simulink model "DSB_LC"  (R2024a)
settings: Solver=VariableStepAuto  StartTime=0.0  StopTime=10.0  RelTol=1e-3
libraries: dspfdesign x1
settings Model: Creator=mohamed
settings SolverCC: AlgebraicLoopSolver=TrustRegion
settings DebuggingCC: UnconnectedInputMsg=warning  UnconnectedOutputMsg=warning  UnconnectedLineMsg=warning
settings ModelReferenceCC: EnableRefExpFcnMdlSchedulingChecks=on
settings SFSimCC: CustomCodeUndefinedFunction=UseInterfaceOnly
settings RTWCC: GPUComputeCapability=3.5  DLArmComputeVersion=19.05

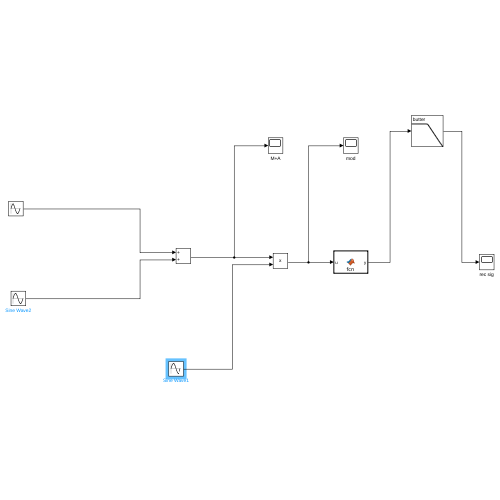
[thumbnail: Simulink's stored preview of the top-level diagram]
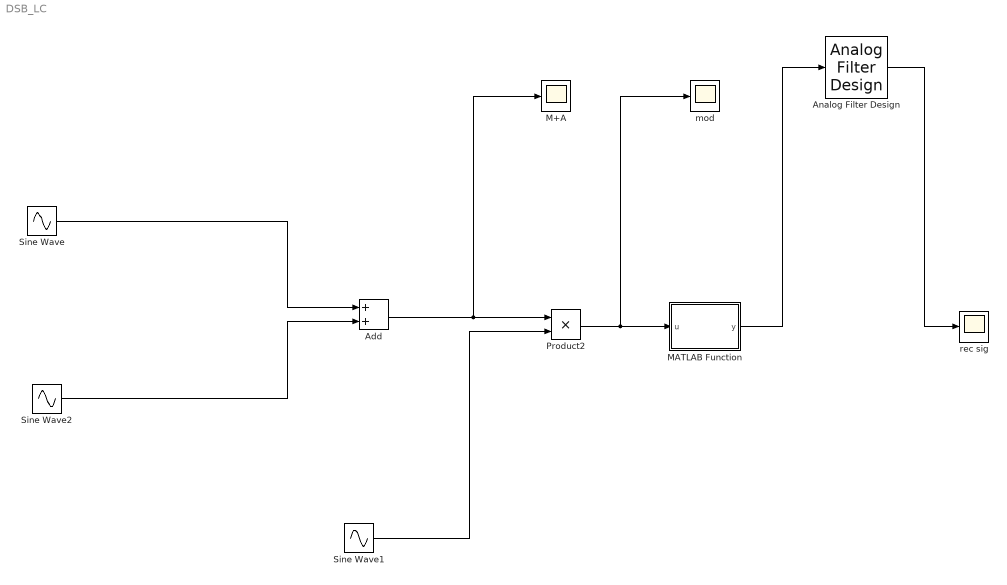
== system DSB_LC ==
  Add : Sum
  Analog Filter Design : dspfdesign/Analog Filter Design  method=Butterworth  filttype=Lowpass  N=8  Wlo=100*pi  Whi=80  Rp=2  Rs=40
  M+A : Scope
  MATLAB Function : MATLAB Function  TreatAsAtomicUnit=on
  Product2 : Product
  Sine Wave : Sin  Amplitude=2  Frequency=10*pi  SampleTime=0
  Sine Wave1 : Sin  Frequency=5000*pi  SampleTime=0
  Sine Wave2 : Sin  Amplitude=3  Frequency=100*pi  Phase=pi/2  SampleTime=0
  mod : Scope
  rec sig : Scope
  wires:
  Sine Wave/1 -> Add/1
  MATLAB Function/1(y) -> Analog Filter Design/1
  Product2/1 -> mod/1, MATLAB Function/1(u)
  Add/1 -> M+A/1, Product2/1
  Sine Wave1/1 -> Product2/2
  Sine Wave2/1 -> Add/2
  Analog Filter Design/1 -> rec sig/1

== matlab function DSB_LC/MATLAB Function ==
  data: u input; y output
function y = fcn(u)
for i=1:length(u)
   if u(i)<0
       u(i)=0;
   end
end
y = u;
